simulink model "PassCarModel_RL_config"  (R2024b)
settings: Solver=FixedStepAuto  StartTime=0.0  StopTime=Tf  FixedStep=.001  RelTol=1e-2
StartFcn:
  | %tic
StopFcn:
  | %toc
model workspace (MAT data in the model file):
  AverageTimeInterval = 0.5
  Downshift_Speeds = [9.5625 12.9375 16.3125 19.6875 23.0625 26.4375 29.8125 33.1875 36.5625 39.9375 43.3125 46.6875 ... (28 elements, 4x7)]
  EEC_Counter : Simulink.Parameter (value not decoded)
  EngRevLim = 7000
  FuzzOffset : Simulink.Parameter (value not decoded)
  FuzzRange : Simulink.Parameter (value not decoded)
  Fuzzing : Simulink.Parameter (value not decoded)
  Pedal_Positions = [0.1 0.4 0.5 0.9]
  TrackPoints = [0 36.336 72.672 109.008 145.344 181.68 218.016 254.352 290.688 327.024 363.36 403.196036522 ... (360 elements, 120x3)]
  Upshift_Speeds = [12.9375 16.3125 19.6875 33 26.4375 29.8125 33.1875 52.5 39.9375 43.3125 46.6875 77.25 ... (28 elements, 4x7)]
  VEH : object (value not decoded)
  gradbp : Simulink.Parameter (value not decoded)
  origin : Simulink.Parameter (value not decoded)
  rayDirections = [0 0 0 0 0 0 0 0 0 0 0 0 ... (363 elements, 121x3)]
  rayLengths = [20 20 20 20 20 20 20 20 20 20 20 20 ... (121 elements, 121x1)]
  rayOrigins = [0.5 0.4 0.3 0.2 0.1 0 -0.1 -0.2 -0.3 -0.4 -0.5 0.5 ... (363 elements, 121x3)]
  theta : Simulink.Parameter (value not decoded)
  totalDistance : Simulink.Parameter (value not decoded)
  vel_profile3 : Simulink.Parameter (value not decoded)
  xEast : Simulink.Parameter (value not decoded)
  yNorth : Simulink.Parameter (value not decoded)
symbols that are objects in the model workspace (value not decoded): gradbp, origin, theta, totalDistance, VEH, vel_profile3, xEast, yNorth
undefined symbols (not defined in the file or in its folder): DecelR, DiscIntNeverNeededParam, dspblkCoreblockFVToolHelper, FO_max, FO_min, FR_max, FR_min, gcbh, ODevR, Sim3dSensor, Ts
libraries: simulink x20, dspstat3 x8, autolibutils x6, sim3dgroundtruthsensorlib x2, rllib x1, slpidlib x1, autolibtranscontrolscommon x1, vehdynlibdriver x1, sharedtransform x1, vehdynlibviscommon x1, vehdynlibsens x1
(part 3 of 5)

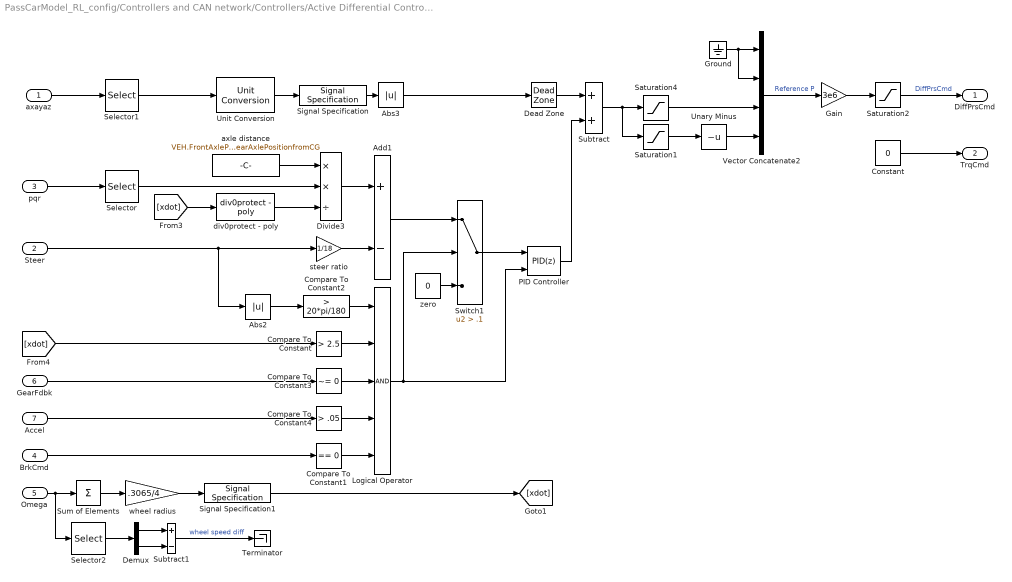
== system PassCarModel_RL_config/Controllers and CAN network/Controllers/Active Differential Control/Rear Diff Controller ==
  axayaz : Inport
  Steer : Inport  Port=2
  pqr : Inport  Port=3
  BrkCmd : Inport  Port=4
  Omega : Inport  Port=5  Unit=rad/s
  GearFdbk : Inport  Port=6
  Accel : Inport  Port=7
  Abs2 : Abs  SaturateOnIntegerOverflow=off
  Abs3 : Abs  ZeroCross=off  SaturateOnIntegerOverflow=off
  Add1 : Sum  Inputs=+-
  Compare To Constant : simulink/Logic and Bit Operations/Compare To Constant  relop=>  const=2.5  OutDataTypeStr=boolean
  Compare To Constant1 : simulink/Logic and Bit Operations/Compare To Constant  relop===  const=0  OutDataTypeStr=boolean
  Compare To Constant2 : simulink/Logic and Bit Operations/Compare To Constant  relop=>  const=20*pi/180  OutDataTypeStr=boolean
  Compare To Constant3 : simulink/Logic and Bit Operations/Compare To Constant  relop=~=  const=0  OutDataTypeStr=boolean
  Compare To Constant4 : simulink/Logic and Bit Operations/Compare To Constant  relop=>  const=.05  OutDataTypeStr=boolean
  Constant : Constant  Value=0
  Dead Zone : DeadZone  ZeroCross=off
  Demux : Demux  Outputs=2
  Divide3 : Product  Inputs=**/
  Gain : Gain  Gain=3e6
  Ground : Ground
  Logical Operator : Logic  Inputs=5  AllPortsSameDT=off  OutDataTypeStr=boolean
  PID Controller : slpidlib/PID Controller  Controller=PID  Form=Parallel  TimeDomain=Discrete-time  UseExternalTs=off  SampleTime=-1  IntegratorMethod=Forward Euler  FilterMethod=Forward Euler  ControllerParametersSource=internal  P=1  I=.05  UseKiTs=off  D=0  UseExternalDerivativeSource=off  N=1  UseFilter=on  TunerSelectOption=Transfer Function Based (PID Tuner App)  ZeroCross=off  InitialConditionSource=internal  InitialConditionForIntegrator=0  InitialConditionForFilter=0  DifferentiatorICPrevScaledInput=0  ExternalReset=either  TrackingMode=off  Kt=1  LimitOutput=on  SatLimitsSource=internal  UpperSaturationLimit=1  LowerSaturationLimit=-1  LinearizeAsGain=on  AntiWindupMode=clamping  Kb=1  LimitIntegrator=off  UpperIntegratorSaturationLimit=inf  LowerIntegratorSaturationLimit=-inf  POutMin=[]  POutMax=[]  IOutMin=[]  IOutMax=[]  DOutMin=[]  DOutMax=[]  NOutMin=[]  NOutMax=[]  SumOutMin=[]  SumOutMax=[]  SaturationOutMin=[]  SaturationOutMax=[]  PParamMin=[]  PParamMax=[]  IParamMin=[]  IParamMax=[]  DParamMin=[]  DParamMax=[]  NParamMin=[]  NParamMax=[]  KbParamMin=[]  KbParamMax=[]  KtParamMin=[]  KtParamMax=[]  KbOutMin=[]  KbOutMax=[]  KtOutMin=[]  KtOutMax=[]  IntegratorOutMin=[]  IntegratorOutMax=[]  FilterOutMin=[]  FilterOutMax=[]  SumI1OutMin=[]  SumI1OutMax=[]  SumI2OutMin=[]  SumI2OutMax=[]  SumI3OutMin=[]  SumI3OutMax=[]  SumI4OutMin=[]  SumI4OutMax=[]  SumDOutMin=[]  SumDOutMax=[]  DifferentiatorOutMin=[]  DifferentiatorOutMax=[]  FilterDiffOutCoefMin=[]  FilterDiffOutCoefMax=[]  ReciprocalOutMin=[]  ReciprocalOutMax=[]  SumDenOutMin=[]  SumDenOutMax=[]  SumNumOutMin=[]  SumNumOutMax=[]  DivideOutMin=[]  DivideOutMax=[]  UdiffTsProdOutMin=[]  UdiffTsProdOutMax=[]  NTsProdOutMin=[]  NTsProdOutMax=[]  UintegralTsProdOutMin=[]  UintegralTsProdOutMax=[]  UngainTsProdOutMin=[]  UngainTsProdOutMax=[]  ClampingZeroOutDataTypeStr=Inherit: Inherit via back propagation  ClampingZeroOutMin=[]  ClampingZeroOutMax=[]  FilterDenConstantOutDataTypeStr=Inherit: Inherit via back propagation  FilterDenConstantOutMin=[]  FilterDenConstantOutMax=[]  PCopyOutDataTypeStr=Inherit: Inherit via back propagation  PCopyOutMin=[]  PCopyOutMax=[]  NCopyOutDataTypeStr=Inherit: Inherit via back propagation  NCopyOutMin=[]  NCopyOutMax=[]  IntegratorContinuousStateAttributes=''  IntegratorStateMustResolveToSignalObject=off  IntegratorRTWStateStorageClass=Auto  FilterContinuousStateAttributes=''  FilterStateMustResolveToSignalObject=off  FilterRTWStateStorageClass=Auto  ParallelPVariant=InternalParameters  IdealPVariant=Disabled  IVariant=InternalParameters  DVariant=InternalParameters  IntegratorVariant=Discrete  SatVariant=Enabled  AWVariant=DiscClampingParallel  PCopyVariant=Disabled  TRVariant=Disabled  FdbkBlocksVariant=Forward  IdealPFdbkVariant=Disabled  SatFdbkVariant=Disabled  DerivativeFilterVariant=ForwardEulerFilter  NVariant=InternalParameters  NCopyVariant=Disabled  FilterICVariant=InternalICsFilter  IntegratorICVariant=InternalICs  ExternalResetVariant=ExternalReset  TRSumVariant=Passthrough  SumFdbkVariant=Disabled  SumVariant=Sum_PID  TsampFilterVariant=InternalTs  TsampNgainVariant=Passthrough  TsampIntegralVariant=Disabled_SignalSpec  ExternalSaturationOutDataTypeStr=Inherit: Same as second input  DerivativeSourceVariant=ErrorSignal  PreIntVariant=InternalPreInt
  Saturation1 : Saturate  UpperLimit=0  LowerLimit=-1  ZeroCross=off
  Saturation2 : Saturate  UpperLimit=5e6  LowerLimit=0  ZeroCross=off
  Saturation4 : Saturate  UpperLimit=1  LowerLimit=0  ZeroCross=off
  Selector : Selector  InputPortWidth=3  IndexOptions=Index vector (dialog)  Indices=[3]  OutputSizes=1
  Selector1 : Selector  InputPortWidth=3  IndexOptions=Index vector (dialog)  Indices=[2]  OutputSizes=1
  Selector2 : Selector  InputPortWidth=4  IndexOptions=Index vector (dialog)  Indices=[3 4]  OutputSizes=1
  Signal Specification : SignalSpecification  Unit=gn
  Signal Specification1 : SignalSpecification  Unit=m/s
  Subtract : Sum
  Subtract1 : Sum  Inputs=+-
  Sum of Elements : Sum  Inputs=+
  Switch1 : Switch  Criteria=u2 > Threshold  Threshold=.1  SaturateOnIntegerOverflow=off  InputSameDT=off
  Terminator : Terminator
  Unary Minus : UnaryMinus
  Unit Conversion : UnitConversion
  Vector Concatenate2 : Concatenate  NumInputs=4
  axle distance : Constant  Value=VEH.FrontAxlePositionfromCG+VEH.RearAxlePositionfromCG
  div0protect - poly : autolibutils/div0protect - poly  thresh=1  ZeroCross1=on  aMode=2
  steer ratio : Gain  Gain=1/18
  wheel radius : Gain  Gain=.3065/4
  zero : Constant  Value=0
  DiffPrsCmd : Outport  VectorParamsAs1DForOutWhenUnconnected=off
  TrqCmd : Outport  Port=2  VectorParamsAs1DForOutWhenUnconnected=off
  wires:
  Vector Concatenate2/1 -> Gain/1  "Reference P"
  Ground/1 -> Vector Concatenate2/2, Vector Concatenate2/1
  Saturation1/1 -> Unary Minus/1
  Gain/1 -> Saturation2/1
  Saturation2/1 -> DiffPrsCmd/1  "DiffPrsCmd"
  Divide3/1 -> Add1/1
  Selector/1 -> Divide3/2
  Logical Operator/1 -> PID Controller/2, Switch1/2
  Switch1/1 -> PID Controller/1
  zero/1 -> Switch1/3
  PID Controller/1 -> Subtract/2
  Add1/1 -> Switch1/1
  axle distance/1 -> Divide3/1
  pqr/1 -> Selector/1
  Compare To Constant2/1 -> Logical Operator/1
  Compare To Constant/1 -> Logical Operator/2
  Abs2/1 -> Compare To Constant2/1
  Steer/1 -> Abs2/1, steer ratio/1
  [xdot] -> Compare To Constant/1
  axayaz/1 -> Selector1/1
  Sum of Elements/1 -> wheel radius/1
  wheel radius/1 -> Signal Specification1/1
  Omega/1 -> Selector2/1, Sum of Elements/1
  Signal Specification1/1 -> [xdot]
  BrkCmd/1 -> Compare To Constant1/1
  GearFdbk/1 -> Compare To Constant3/1
  Compare To Constant3/1 -> Logical Operator/3
  Subtract/1 -> Saturation1/1, Saturation4/1
  Accel/1 -> Compare To Constant4/1
  Compare To Constant4/1 -> Logical Operator/4
  steer ratio/1 -> Add1/2
  Saturation4/1 -> Vector Concatenate2/3
  Selector1/1 -> Unit Conversion/1
  Signal Specification/1 -> Abs3/1
  Abs3/1 -> Dead Zone/1
  Dead Zone/1 -> Subtract/1
  Constant/1 -> TrqCmd/1
  Selector2/1 -> Demux/1
  Demux/1 -> Subtract1/1
  Demux/2 -> Subtract1/2
  Unary Minus/1 -> Vector Concatenate2/4
  Subtract1/1 -> Terminator/1  "wheel speed diff"
  Compare To Constant1/1 -> Logical Operator/5
  Unit Conversion/1 -> Signal Specification/1
  [xdot] -> div0protect - poly/1
  div0protect - poly/1 -> Divide3/3

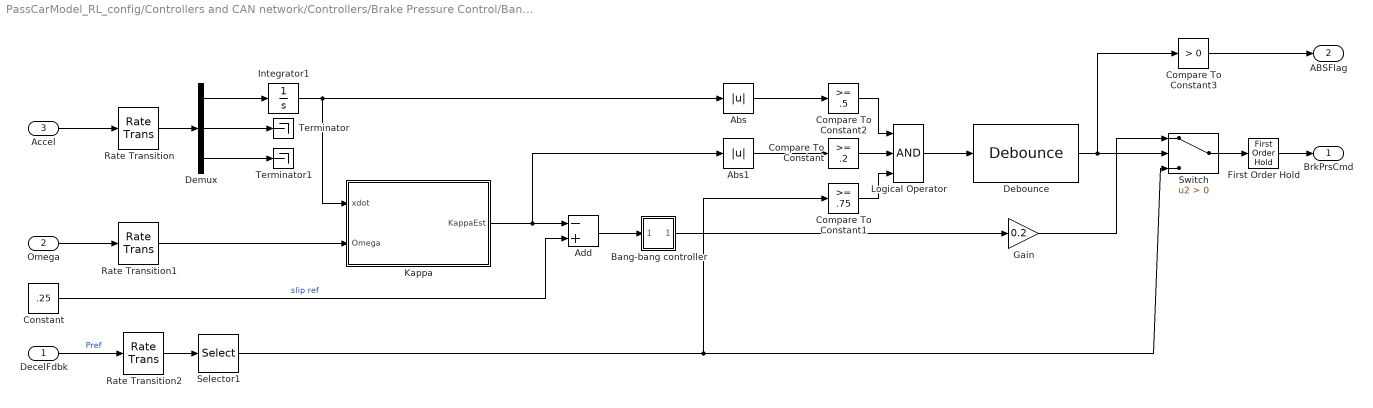
== system PassCarModel_RL_config/Controllers and CAN network/Controllers/Brake Pressure Control/Bang Bang ABS ==
  DecelFdbk : Inport
  Omega : Inport  Port=2
  Accel : Inport  Port=3
  Abs : Abs  SaturateOnIntegerOverflow=off
  Abs1 : Abs  SaturateOnIntegerOverflow=off
  Add : Sum  Inputs=-+
  Bang-bang controller : Subsystem  mask(Sign){}
      mask help: y = sign(x)
      mask Help: Sign Function:\n\t\t\ty = 1 if x > 0\n\t\t\ty = 0 if x = 0\n\t\t\ty = -1 if x < 0
      mask Display: plot(-50,-50,50,50,[-50,50],[0,0],[0,0],[-50,50],[-40,0],[-30,-30],[0,40],[30,30])
  Compare To Constant : simulink/Logic and Bit Operations/Compare To Constant  relop=>=  const=.2  OutDataTypeStr=boolean
  Compare To Constant1 : simulink/Logic and Bit Operations/Compare To Constant  relop=>=  const=.75  OutDataTypeStr=boolean
  Compare To Constant2 : simulink/Logic and Bit Operations/Compare To Constant  relop=>=  const=.5  OutDataTypeStr=boolean
  Compare To Constant3 : simulink/Logic and Bit Operations/Compare To Constant  relop=>  const=0  OutDataTypeStr=boolean  ZeroCross=off
  Constant : Constant  Value=.25
  Debounce : autolibutils/Debounce  DbcOn_Cnts=.1*.001  DbcOff_Cnts=.1*.001  aMode=2
  Demux : Demux  Outputs=3
  First Order Hold : FirstOrderHold  ErrorTolerance=1
  Gain : Gain  Gain=0.2
  Integrator1 : Integrator
  Kappa : Subsystem  TreatAsAtomicUnit=on
  Logical Operator : Logic  Inputs=3  AllPortsSameDT=off  OutDataTypeStr=boolean
  Rate Transition : RateTransition  Deterministic=off  OutPortSampleTime=.001
  Rate Transition1 : RateTransition  Deterministic=off  OutPortSampleTime=.001
  Rate Transition2 : RateTransition  Deterministic=off  OutPortSampleTime=.001
  Selector1 : Selector  InputPortWidth=1  IndexOptions=Index vector (dialog)  Indices=[1 1 1 1]  OutputSizes=1
  Switch : Switch  Criteria=u2 > Threshold  ZeroCross=off  SaturateOnIntegerOverflow=off  InputSameDT=off
  Terminator : Terminator
  Terminator1 : Terminator
  BrkPrsCmd : Outport  VectorParamsAs1DForOutWhenUnconnected=off
  ABSFlag : Outport  Port=2
  wires:
  Bang-bang controller/1(out_1) -> Gain/1
  Add/1 -> Bang-bang controller/1(in_1)
  First Order Hold/1 -> BrkPrsCmd/1
  DecelFdbk/1 -> Rate Transition2/1  "Pref"
  Constant/1 -> Add/2  "slip ref"
  Switch/1 -> First Order Hold/1
  Kappa/1(KappaEst) -> Add/1, Abs1/1
  Logical Operator/1 -> Debounce/1
  Compare To Constant/1 -> Logical Operator/2
  Compare To Constant1/1 -> Logical Operator/3
  Debounce/1 -> Compare To Constant3/1, Switch/2
  Abs/1 -> Compare To Constant2/1
  Compare To Constant2/1 -> Logical Operator/1
  Gain/1 -> Switch/1
  Integrator1/1 -> Kappa/1(xdot), Abs/1
  Demux/2 -> Terminator/1
  Accel/1 -> Rate Transition/1
  Demux/1 -> Integrator1/1
  Rate Transition/1 -> Demux/1
  Demux/3 -> Terminator1/1
  Omega/1 -> Rate Transition1/1
  Rate Transition1/1 -> Kappa/2(Omega)
  Rate Transition2/1 -> Selector1/1
  Compare To Constant3/1 -> ABSFlag/1
  Selector1/1 -> Compare To Constant1/1, Switch/3
  Abs1/1 -> Compare To Constant/1

== system PassCarModel_RL_config/Controllers and CAN network/Controllers/Brake Pressure Control/Five-State ABS and TCS ==
  note: The first order hold block behaves strange: it keeps the ABS flag non-zero after the ABS operation. Its check (if ABS is active) fails elsewhere.
      |
      | The the block is removed
  note: The first order hold block behaves strange: it keeps the ABS flag non-zero after the ABS operation. Its check (if ABS is active) fails elsewhere.
      |
      | The the block is removed
  DecelFdbk : Inport
  Omega : Inport  Port=2
  Accel : Inport  Port=3
  AccelFdbk : Inport  Port=4
  BrkPrs : Inport  Port=5
  ABSCtrlForEach : Subsystem  mask(Five-State ABS Control){Re=0.323, KappaOpt=-0.12, WhlAccelOpt=[-9.8,-9.8,-20,-20], v1=0, v5=0.55, v4=1, a2=-1.5, b=-1.5, A=4.5, a1=3.6, aMode=2}
      mask prompts: Re "Wheel effective radius, Re [m]:"; KappaOpt "Desired wheel slip ratio, KappaOpt [-]:"; WhlAccelOpt "Desired wheel acceleration, WhlAccelOpt [m/s^2]:"; v1 "Braking realease command, v1 [-]:"; v5 "Braking hold command, v5 [-]:"; v4 "Braking add command, v4 [-]:"; a2 "Threshold of State 1, a2 [m/s^2]:"; b "Threshold of State 2, b [m/s^2]:"; A "Threshold of State 3 and 4, A [m/s^2]:"; a1 "Threshold of State 5, a1 [m/s^2]:"
      mask help: This block determines brake pressure varying rate for each wheel once the ABS controller is activated. During ABS control, only wheel speed is directly regulated.
      mask init:
      | [~]=vehdynicon('vehdynblk',gcb);
      mask DialogControl vehParamGroup Prompt: Vehicle Parameter
      mask DialogControl ParameterGroupVar Prompt: Desired Control Parameters
      mask DialogControl Container3 Prompt: Braking Pressure Rates
      mask DialogControl Container4 Prompt: Wheel Acceleration Thresholds
  First Order Hold : FirstOrderHold  ErrorTolerance=.001  AllowContinuousInput=on
  Logical Operator : Logic  Operator=OR  AllPortsSameDT=off  OutDataTypeStr=boolean
  Sum : Sum  Inputs=|++
  Switch : Switch  Criteria=u2 > Threshold  SaturateOnIntegerOverflow=off  InputSameDT=off
  TCSCtrlForEach : Subsystem  mask(Five-State TCS Control){Re=0.323, KappaOpt=0.12, WhlAccelOpt=[11, 11, 11, 11], v1=1.5, v5=-0.5, v4=-1.2, a2=-3, b=-10, A=-11, a1=-9, aMode=2}
      mask prompts: Re "Wheel effective radius, Re [m]:"; KappaOpt "Desired wheel slip ratio, KappaOpt [-]:"; WhlAccelOpt "Desired wheel acceleration, WhlAccelOpt [m/s^2]:"; v1 "Braking pressure rising rate, v1 [-]:"; v5 "Secondary braking pressure declining rate, v5 [-]:"; v4 "Braking pressure declining rate, v4 [-]:"; a2 "Threshold of State 1, a2 [m/s^2]:"; b "Threshold of State 2, b [m/s^2]:"; A "Threshold of State 3 and 4, A [m/s^2]:"; a1 "Threshold of State 5, a1 [m/s^2]:"
      mask help: This block determines brake pressure varying rate for each wheel once the TCS controller is activated. During TCS control, only wheel speed is directly regulated.
      mask init:
      | [~]=vehdynicon('vehdynblk',gcb);
      mask DialogControl vehParamGroup Prompt: Vehicle Parameter
      mask DialogControl ParameterGroupVar Prompt: Desired Control Parameters
      mask DialogControl Container3 Prompt: Braking Pressure Rates
      mask DialogControl Container4 Prompt: Wheel Acceleration Thresholds
  Wheel Accel and Slip Estimator : Subsystem
  BrkPrsCmd : Outport
  ABSFlag : Outport  Port=2  PortDimensions=4
  TCSFlag : Outport  Port=3  PortDimensions=4
  wires:
  Wheel Accel and Slip Estimator/1(<WhlAccel>) -> TCSCtrlForEach/1(WhlAccel), ABSCtrlForEach/2(WhlAccel)
  Wheel Accel and Slip Estimator/2(<Kappa>) -> TCSCtrlForEach/2(WhlSlip), ABSCtrlForEach/3(WhlSlip)
  Wheel Accel and Slip Estimator/3(<xdot>) -> ABSCtrlForEach/4(VehSpd)
  First Order Hold/1 -> BrkPrsCmd/1
  ABSCtrlForEach/2(BrkFlag) -> ABSFlag/1, Logical Operator/1
  Switch/1 -> First Order Hold/1
  TCSCtrlForEach/2(BrkFlag) -> TCSFlag/1, Logical Operator/2
  TCSCtrlForEach/1(BrkCtrl) -> Sum/2
  ABSCtrlForEach/1(BrkCtrl) -> Sum/1
  Sum/1 -> Switch/1
  Logical Operator/1 -> Switch/2
  Accel/1 -> Wheel Accel and Slip Estimator/2(Accel)
  DecelFdbk/1 -> Switch/3, ABSCtrlForEach/1(Pref)
  Omega/1 -> Wheel Accel and Slip Estimator/1(Omega)
  AccelFdbk/1 -> TCSCtrlForEach/3(AccelFdbk)
  BrkPrs/1 -> TCSCtrlForEach/4(PbFdbk)

== system PassCarModel_RL_config/Controllers and CAN network/Controllers/Brake Pressure Control/Open Loop ==
  DecelFdbk : Inport
  Constant : Constant  Value=false
  Constant1 : Constant  Value=false
  Selector : Selector  InputPortWidth=1  IndexOptions=Index vector (dialog)  Indices=[1 1 1 1]  OutputSizes=1
  Selector1 : Selector  InputPortWidth=1  IndexOptions=Index vector (dialog)  Indices=[1 1 1 1]  OutputSizes=1
  Selector2 : Selector  InputPortWidth=1  IndexOptions=Index vector (dialog)  Indices=[1 1 1 1]  OutputSizes=1
  BrkPrsCmd : Outport  VectorParamsAs1DForOutWhenUnconnected=off
  ABSFlag : Outport  Port=2
  TCSFlag : Outport  Port=3
  wires:
  DecelFdbk/1 -> Selector1/1
  Selector1/1 -> BrkPrsCmd/1
  Constant/1 -> Selector/1
  Selector/1 -> ABSFlag/1
  Selector2/1 -> TCSFlag/1
  Constant1/1 -> Selector2/1

== system PassCarModel_RL_config/Controllers and CAN network/Controllers/Brake Pressure Control/Slip control ==
  DecelFdbk : Inport
  Omega : Inport  Port=2
  Accel : Inport  Port=3
  AccelFdbk : Inport  Port=4
  BrkPrs : Inport  Port=5
  ABSCtrlForEach : Subsystem  SystemSampleTime=0.005  mask(Five-State ABS Control){KappaOpt=0, v1=0, v5=0.55, v3=1, a0=-0.5, a1=-0.2, a2=-0.2, a3=-0.05, a4=-0.2, a5=-0.15}
      mask prompts: KappaOpt "Desired wheel slip ratio, KappaOpt [-]:"; v1 "Braking realease command, v1 [-]:"; v5 "Braking hold command, v5 [-]:"; v3 "Braking add command, v3 [-]:"; a0 "Threashold of ABS activation, a0 [-]:"; a1 "Threshold of State 1, a1 [-]:"; a2 "Threshold of State 2, a2 [-]:"; a3 "Threshold of State 3, a3 [-]:"; a4 "Threshold of State 4, a4 [-]:"; a5 "Threshold of State 5, a5 [-]:"
      mask help: This block determines brake pressure varying rate for each wheel once the ABS controller is activated. During ABS control, only wheel speed is directly regulated.
      mask init:
      | [~]=vehdynicon('vehdynblk',gcb);
      mask DialogControl ParameterGroupVar Prompt: Desired Control Parameters
      mask DialogControl Container3 Prompt: Braking Pressure Rates
      mask DialogControl Container4 Prompt: Wheel Slip Thresholds
  First Order Hold : FirstOrderHold  ErrorTolerance=.01  AllowContinuousInput=on
  Logical Operator : Logic  Operator=OR  AllPortsSameDT=off  OutDataTypeStr=boolean
  Sum : Sum  Inputs=|++
  Switch : Switch  Criteria=u2 > Threshold  SaturateOnIntegerOverflow=off  InputSameDT=off
  TCSCtrlForEach : Subsystem  mask(Five-State TCS Control){Re=0.323, KappaOpt=0.12, WhlAccelOpt=[11, 11, 11, 11], v1=1.5, v5=-0.5, v4=-1.2, a2=-6, b=-10, A=-11, a1=-9, aMode=2}
      mask prompts: Re "Wheel effective radius, Re [m]:"; KappaOpt "Desired wheel slip ratio, KappaOpt [-]:"; WhlAccelOpt "Desired wheel acceleration, WhlAccelOpt [m/s^2]:"; v1 "Braking pressure rising rate, v1 [-]:"; v5 "Secondary braking pressure declining rate, v5 [-]:"; v4 "Braking pressure declining rate, v4 [-]:"; a2 "Threshold of State 1, a2 [m/s^2]:"; b "Threshold of State 2, b [m/s^2]:"; A "Threshold of State 3 and 4, A [m/s^2]:"; a1 "Threshold of State 5, a1 [m/s^2]:"
      mask help: This block determines brake pressure varying rate for each wheel once the TCS controller is activated. During TCS control, only wheel speed is directly regulated.
      mask init:
      | [~]=vehdynicon('vehdynblk',gcb);
      mask DialogControl vehParamGroup Prompt: Vehicle Parameter
      mask DialogControl ParameterGroupVar Prompt: Desired Control Parameters
      mask DialogControl Container3 Prompt: Braking Pressure Rates
      mask DialogControl Container4 Prompt: Wheel Acceleration Thresholds
  Wheel Accel and Slip Estimator : Subsystem
  ABSFlag : Outport
  BrkPrsCmd : Outport  Port=2
  TCSFlag : Outport  Port=3
  wires:
  TCSCtrlForEach/2(BrkFlag) -> TCSFlag/1, Logical Operator/2
  Wheel Accel and Slip Estimator/1(<WhlAccel>) -> TCSCtrlForEach/1(WhlAccel)
  ABSCtrlForEach/2(BrkFlag) -> ABSFlag/1, Logical Operator/1
  ABSCtrlForEach/1(BrkCtrl) -> Sum/1
  TCSCtrlForEach/1(BrkCtrl) -> Sum/2
  Switch/1 -> First Order Hold/1
  First Order Hold/1 -> BrkPrsCmd/1
  Wheel Accel and Slip Estimator/2(<Kappa>) -> TCSCtrlForEach/2(WhlSlip), ABSCtrlForEach/2(WhlSlip)
  Omega/1 -> Wheel Accel and Slip Estimator/1(Omega)
  DecelFdbk/1 -> Switch/3, ABSCtrlForEach/1(Pref)
  Sum/1 -> Switch/1
  AccelFdbk/1 -> TCSCtrlForEach/3(AccelFdbk)
  Wheel Accel and Slip Estimator/3(<xdot>) -> ABSCtrlForEach/3(VehSpd)
  BrkPrs/1 -> TCSCtrlForEach/4(PbFdbk)
  Logical Operator/1 -> Switch/2
  Accel/1 -> Wheel Accel and Slip Estimator/2(Accel)

== system PassCarModel_RL_config/Controllers and CAN network/Controllers/ECU/Torque Cmd ==
  note: ABSFlag is a vector of 4 (number of wheels
      | each element should be an integer in [0..5],
      | however it can be a small number instead of zero
  DiffTrqCmd : Inport
  <Accel> : Inport  Port=2
  EngSpd : Inport  Port=3
  ABSFlag : Inport  Port=4
  Acc to Torque Request : Gain  Gain=150
  Constant : Constant  Value=0
  Max : MinMax  Function=max  Inputs=2
  Max of Elements : MinMax  Function=max
  Rev Limiter Control : Subsystem
  Signal Specification : SignalSpecification  Unit=rpm
  Switch : Switch  Criteria=u2 > Threshold  Threshold=0.1  ZeroCross=off  SaturateOnIntegerOverflow=off  InputSameDT=off
  Unit Conversion : UnitConversion
  EngTrqCmd : Outport
  wires:
  Signal Specification/1 -> Rev Limiter Control/2(EngSpd)  "EngSpd"
  Unit Conversion/1 -> Signal Specification/1
  EngSpd/1 -> Unit Conversion/1
  <Accel>/1 -> Acc to Torque Request/1
  Acc to Torque Request/1 -> Rev Limiter Control/1(TrqCmd)
  DiffTrqCmd/1 -> Max/1
  Rev Limiter Control/1(TrqCmdRevLimited) -> Max/2
  Switch/1 -> EngTrqCmd/1
  Max/1 -> Switch/3
  ABSFlag/1 -> Max of Elements/1
  Constant/1 -> Switch/1
  Max of Elements/1 -> Switch/2

== system PassCarModel_RL_config/Controllers and CAN network/Controllers/Transmission Controller/Driver - No Clutch ==
  GearReq : Inport
  Gear : Outport  VectorParamsAs1DForOutWhenUnconnected=off
  wires:
  GearReq/1 -> Gear/1

== system PassCarModel_RL_config/Controllers and CAN network/Controllers/Transmission Controller/PRNDL Controller ==
  Accel : Inport
  BrkCmd : Inport  Port=2
  Omega : Inport  Port=3  Unit=rad/s
  EngSpd : Inport  Port=4  Unit=rad/s
  GearReq : Inport  Port=5
  ABSFlag : Inport  Port=6
  Gain : Gain  Gain=.3065/4
  Logical Operator : Logic  Operator=OR  Inputs=1  AllPortsSameDT=off  OutDataTypeStr=boolean
  Signal Specification1 : SignalSpecification  Unit=m/s
  Sum of Elements : Sum  Inputs=+
  Transmission Controller PRNDL : autolibtranscontrolscommon/Transmission Controller PRNDL  DriveMode=off  GearInit=1  LugSpd=1200  MinUpSpd=2000  tClutchUp=0.5  tClutchDn=0.5  tPark=120  VelUnit=km/hr  UpShSpd="reshape([20    25    30    45    35    45    40    55    40    55    55    65    50    60    65    75    60    65    80    90    70    75   120   150    85    85   150   185  20    25    30    45    35    45    40    55    40    55    55    65    50    60    65    75    60    65    80    90    70    75   120   150    85    85   150   185],4,7,2)"  UpLdBpt=[.1 .4 .75 1]  UpShBpt=1:7  UpPtBpt=[1 2]  DnShfSpd="reshape([10    10    12    15    15    18    18    20    25    25    21    25    30    35    55    55    40    50    65    70    55    65    75    80    75    80    85    95   10    10    12    15    15    18    18    20    25    25    21    25    30    35    55    55    40    50    65    70    55    65    75    80    75    80    85    95],4,7,2)"  DnShSpd=[10 15 25 30 40 55 75; 10 18 25 35 50 65 80; 12 18 21 55 65 75 85; 15 20 25 55 70 80 95]  DnLdBpt=[.1 .4 .75 1]  DnShBpt=2:8  DnPtBpt=[1 2]  POFS=zeros(4,1)  GOFS=zeros(1,7)  Ngears=8  aMode=2
  Gear : Outport  VectorParamsAs1DForOutWhenUnconnected=off
  wires:
  Gain/1 -> Signal Specification1/1
  Omega/1 -> Sum of Elements/1
  Sum of Elements/1 -> Gain/1
  ABSFlag/1 -> Logical Operator/1
  Transmission Controller PRNDL/1 -> Gear/1
  GearReq/1 -> Transmission Controller PRNDL/1  "PRNDL"
  Accel/1 -> Transmission Controller PRNDL/2
  BrkCmd/1 -> Transmission Controller PRNDL/3
  Signal Specification1/1 -> Transmission Controller PRNDL/4
  EngSpd/1 -> Transmission Controller PRNDL/5
  Logical Operator/1 -> Transmission Controller PRNDL/6

== system PassCarModel_RL_config/Controllers and CAN network/Controllers/Transmission Controller/Paddles ==
  Accel : Inport
  EngSpd : Inport  Port=2  Unit=rad/s
  Add1 : Sum  Inputs=+-+
  Current Gear : UnitDelay  SampleTime=-1  HasFrameUpgradeWarning=on
  Data Type Conversion2 : DataTypeConversion  OutDataTypeStr=double  SaturateOnIntegerOverflow=off  RndMeth=Floor
  Debounce : autolibutils/Debounce  DbcOn_Cnts=10  DbcOff_Cnts=10  aMode=aMode
  Debounce1 : autolibutils/Debounce  DbcOn_Cnts=10  DbcOff_Cnts=10  aMode=aMode
  Demux : Demux  Outputs=2
  Detect Increase2 : simulink/Logic and Bit Operations/Detect Increase  vinit=0.0  OutDataTypeStr=boolean
  Logical Operator1 : Logic  Operator=XOR  Inputs=1  AllPortsSameDT=off  OutDataTypeStr=boolean
  Mux : Mux  Inputs=2
  Switch2 : Switch  Criteria=u2 > Threshold  SaturateOnIntegerOverflow=off  InputSameDT=off
  Gear : Outport  VectorParamsAs1DForOutWhenUnconnected=off
  wires:
  Debounce/1 -> Mux/1
  Mux/1 -> Detect Increase2/1
  Logical Operator1/1 -> Switch2/2
  Data Type Conversion2/1 -> Demux/1
  Demux/1 -> Add1/1
  Demux/2 -> Add1/2
  Current Gear/1 -> Add1/3, Switch2/3
  Switch2/1 -> Gear/1, Current Gear/1
  Debounce1/1 -> Mux/2
  Add1/1 -> Switch2/1
  Detect Increase2/1 -> Data Type Conversion2/1, Logical Operator1/1
  EngSpd/1 -> Debounce1/1
  Accel/1 -> Debounce/1

== system PassCarModel_RL_config/Controllers and CAN network/Controllers/Transmission Controller/Transmission Controller ==
  Accel : Inport
  EngSpd : Inport  Port=2  Unit=rad/s
  Omega : Inport  Port=3  Unit=rad/s
  10ms Function-Call Generator : simulink/Ports & Subsystems/Function-Call Generator  sample_time=0.01  numberOfIterations=1  DisallowWideOutput=off
  Data Type Conversion : DataTypeConversion  SaturateOnIntegerOverflow=off  RndMeth=Floor
  First Order Hold : FirstOrderHold  ErrorTolerance=.1
  Rate Transition : RateTransition  Deterministic=off
  Rate Transition1 : RateTransition  Deterministic=off
  Rate Transition2 : RateTransition  Deterministic=off
  Signal Specification : SignalSpecification  Unit=rpm
  TCM : Subsystem
  Unit Conversion : UnitConversion
  Gear : Outport  VectorParamsAs1DForOutWhenUnconnected=off
  wires:
  TCM/1(GearCmd) -> Data Type Conversion/1
  Rate Transition/1 -> TCM/1(AccCmd)
  10ms Function-Call Generator/1 -> TCM/Trigger
  Accel/1 -> Rate Transition/1
  Omega/1 -> Rate Transition2/1
  Rate Transition1/1 -> TCM/2(EngSpd)
  First Order Hold/1 -> Gear/1
  Unit Conversion/1 -> Signal Specification/1
  Signal Specification/1 -> Rate Transition1/1  "EngSpd"
  EngSpd/1 -> Unit Conversion/1
  Data Type Conversion/1 -> First Order Hold/1
  Rate Transition2/1 -> TCM/3(Omega)

== system PassCarModel_RL_config/Controllers and CAN network/Gateway/BC-Filter/FilterABSTCSFlags ==
  In1 : Inport
  In2 : Inport  Port=2
  Out1 : Outport
  Out2 : Outport  Port=2
  wires:
  In1/1 -> Out1/1
  In2/1 -> Out2/1

== system PassCarModel_RL_config/Controllers and CAN network/Gateway/BC-Filter/FilterBrkPrs ==
  In1 : Inport
  Out1 : Outport
  wires:
  In1/1 -> Out1/1

== system PassCarModel_RL_config/Controllers and CAN network/Gateway/BC-Filter/FilterBrkPrsCmd ==
  In1 : Inport
  Out1 : Outport
  wires:
  In1/1 -> Out1/1

== system PassCarModel_RL_config/Controllers and CAN network/Gateway/BC-Filter/FilterWheelSpeed ==
  VehicleSpeed : Inport
  Omega : Inport  Port=2
  PrpShftSpd : Inport  Port=3
  OmegaFuzz : Inport  Port=4
  AllCombinationCounted : Subsystem
  Bus Creator : BusCreator  Inputs=4
  Data Type Conversion : DataTypeConversion  SaturateOnIntegerOverflow=off  RndMeth=Floor
  Data Type Conversion{1..7} (7 alike) : DataTypeConversion  OutDataTypeStr=double  SaturateOnIntegerOverflow=off  RndMeth=Floor
  MATLAB Function : MATLAB Function  TreatAsAtomicUnit=on
  Signal holder : Subsystem
  Terminator{,2..5} (5 alike) : Terminator
  OmegaFiltered : Outport
  wires:
  MATLAB Function/2(diff_ratio) -> Data Type Conversion3/1  "diff_ratio"
  MATLAB Function/4(y1) -> Data Type Conversion5/1  "RearAxle_WS_check"
  MATLAB Function/1(y) -> Data Type Conversion7/1  "Decision"
  MATLAB Function/3(wheel_speed_max) -> Data Type Conversion4/1  "wheel_speed_max"
  MATLAB Function/5(y2) -> Data Type Conversion6/1  "VehSpeed_WS_Check"
  VehicleSpeed/1 -> Data Type Conversion/1
  PrpShftSpd/1 -> Data Type Conversion1/1
  OmegaFuzz/1 -> AllCombinationCounted/2(Input2)
  AllCombinationCounted/2(Input1 && ~Input2) -> Bus Creator/2  "RealAccept"
  AllCombinationCounted/1(Input1 && Input2) -> Bus Creator/1  "FuzzAccept"
  AllCombinationCounted/3(~Input1 && Input2) -> Bus Creator/3  "FuzzReject"
  AllCombinationCounted/4(~Input1 && ~Input2) -> Bus Creator/4  "RealReject"
  Bus Creator/1 -> Terminator/1  "FilterEfficiency"
  Omega/1 -> Data Type Conversion2/1, Signal holder/1(SignalIn)  "OmegaRaw"
  Signal holder/1(SignalOut) -> OmegaFiltered/1  "OmegaFiltered"
  Data Type Conversion/1 -> MATLAB Function/3(VehSpeed)
  Data Type Conversion1/1 -> MATLAB Function/2(OutputShaftSpeed)
  Data Type Conversion2/1 -> MATLAB Function/1(WheelSpeeds)
  Data Type Conversion3/1 -> Terminator2/1
  Data Type Conversion4/1 -> Terminator3/1
  Data Type Conversion5/1 -> Terminator4/1
  Data Type Conversion6/1 -> Terminator5/1
  Data Type Conversion7/1 -> AllCombinationCounted/1(Input1), Signal holder/2(Condition)

== system PassCarModel_RL_config/Vehicle with driver and environment/Environment/Ground Feedback/3D Engine ==
  Friction : Inport
  VehFdbk : Inport  Port=2
  3D Engine Source : Subsystem  Variant=on  VariantControl=Choice  mask(Terrain Source){terrType=Single point}
      mask prompts: terrType "Terrain feedback type:"
      mask help:
      | This variant subsystem provides the option for:
      | - a single point of contact for each wheel with minimal post-processing ideal for smooth surfaces and maximum run-time performance.
      | - multiple points of contact per wheel which may be used when interested in non-smooth terrain at a higher computational cost.
      mask TypeOptions terrType: Single point | Multiple points
  Bus Creator2 : BusCreator  Inputs=4
  Bus Creator3 : BusCreator  Inputs=3
  Demux1 : Demux
  Signal Specification1 : SignalSpecification  Unit=1
  Ground : Outport  VectorParamsAs1DForOutWhenUnconnected=off
  wires:
  Signal Specification1/1 -> Demux1/1
  Demux1/1 -> Bus Creator2/1  "mu_FL"
  Demux1/3 -> Bus Creator2/3  "mu_RL"
  Demux1/4 -> Bus Creator2/4  "mu_RR"
  Demux1/2 -> Bus Creator2/2  "mu_FR"
  Bus Creator2/1 -> Bus Creator3/3  "mu"
  Bus Creator3/1 -> Ground/1
  Friction/1 -> Signal Specification1/1
  VehFdbk/1 -> 3D Engine Source/1(VehFdbk)
  3D Engine Source/1(z) -> Bus Creator3/1  "z"
  3D Engine Source/2(DCM) -> Bus Creator3/2  "DCM"

== system PassCarModel_RL_config/Vehicle with driver and environment/Environment/Ground Feedback/Constant ==
  Friction : Inport
  Bus Creator : BusCreator  Inputs=4
  Bus Creator2 : BusCreator  Inputs=4
  Bus Creator3 : BusCreator  Inputs=3
  Constant1 : Constant  Value=zeros(4,1)
  Constant4 : Constant  Value=repmat(eye(3),1,1,4)
  Demux : Demux
  Demux1 : Demux
  Signal Specification : SignalSpecification  Unit=m
  Signal Specification1 : SignalSpecification  Unit=1
  Ground : Outport  VectorParamsAs1DForOutWhenUnconnected=off
  wires:
  Constant1/1 -> Signal Specification/1
  Signal Specification/1 -> Demux/1
  Demux/4 -> Bus Creator/4  "G_RR_z"
  Demux/1 -> Bus Creator/1  "G_FL_z"
  Demux/3 -> Bus Creator/3  "G_RL_z"
  Demux/2 -> Bus Creator/2  "G_FR_z"
  Bus Creator/1 -> Bus Creator3/1  "z"
  Demux1/3 -> Bus Creator2/3  "mu_RL"
  Demux1/4 -> Bus Creator2/4  "mu_RR"
  Demux1/1 -> Bus Creator2/1  "mu_FL"
  Demux1/2 -> Bus Creator2/2  "mu_FR"
  Bus Creator2/1 -> Bus Creator3/3  "mu"
  Friction/1 -> Signal Specification1/1
  Signal Specification1/1 -> Demux1/1
  Bus Creator3/1 -> Ground/1
  Constant4/1 -> Bus Creator3/2  "DCM"

== system PassCarModel_RL_config/Vehicle with driver and environment/Environment/Road Track Friction/2D Lookup Tbl for Scaling Fctr (Lambda) ==
  XWhl : Inport  Partition=on  PartitionDimension=1  PartitionWidth=1  PartitionOffset=0
  YWhl : Inport  Port=2  Partition=on  PartitionDimension=1  PartitionWidth=1  PartitionOffset=0
  XBpt : Inport  Port=3
  YBpt : Inport  Port=4
  2-D Lookup Table : Lookup_n-D  BreakpointsForDimension1Source=Input port  BreakpointsForDimension1=xbr  BreakpointsForDimension2Source=Input port  BreakpointsForDimension2=ybr  BeginIndexSearchUsingPreviousIndexResult=on  Table=mutable  ExtrapMethod=Clip  InternalRulePriority=Speed  RndMeth=Simplest
      settings: InputPortMap=u0,u1,p5,p7
  For Each : ForEach  DisableCoverage=on
  Lambda for each whl : Outport  ConcatenationDimension=1
  wires:
  XWhl/1 -> 2-D Lookup Table/1
  YWhl/1 -> 2-D Lookup Table/2
  2-D Lookup Table/1 -> Lambda for each whl/1
  XBpt/1 -> 2-D Lookup Table/3
  YBpt/1 -> 2-D Lookup Table/4

== system PassCarModel_RL_config/Vehicle with driver and environment/Environment/Road Track Friction/Creating Inertial Frm Bpt ==
  XCg : Inport
  YCg : Inport  Port=2
  Enable : EnablePort
  Add : Sum
  Add1 : Sum
  Constant1 : Constant  Value=ybr
  Constant3 : Constant  Value=xbr
  XBpt : Outport
  YBpt : Outport  Port=2
  wires:
  Add/1 -> XBpt/1
  Constant1/1 -> Add1/1
  Add1/1 -> YBpt/1
  Constant3/1 -> Add/2
  YCg/1 -> Add1/2
  XCg/1 -> Add/1

== system PassCarModel_RL_config/Vehicle with driver and environment/Environment/Road Track Friction/En at t = 0 ==
  Clock1 : Clock
  Compare To Zero : simulink/Logic and Bit Operations/Compare To Zero  relop===  OutDataTypeStr=boolean
  Constant : Constant
  Constant2 : Constant  Value=0
  Switch1 : Switch  Criteria=u2 > Threshold  SaturateOnIntegerOverflow=off  InputSameDT=off
  Out1 : Outport
  wires:
  Clock1/1 -> Compare To Zero/1
  Constant2/1 -> Switch1/3
  Constant/1 -> Switch1/1
  Switch1/1 -> Out1/1
  Compare To Zero/1 -> Switch1/2

== system PassCarModel_RL_config/Vehicle with driver and environment/Passenger Vehicle/Pedal Cluster and Cabin/Brake Pedal ==
  DecelCmd : Inport
  Constant1 : Constant  Value=-20
  Dead Zone1 : DeadZone  LowerValue=0  UpperValue=.01  ZeroCross=off
  Gain3 : Gain  Gain=40
  Integrator2 : Integrator  LimitOutput=on  UpperSaturationLimit=1  LowerSaturationLimit=0
  Switch1 : Switch  Criteria=u2 > Threshold  Threshold=.1  SaturateOnIntegerOverflow=off  InputSameDT=off
  DecelFdbk : Outport
  wires:
  Dead Zone1/1 -> Switch1/2, Gain3/1
  Constant1/1 -> Switch1/3
  Integrator2/1 -> DecelFdbk/1
  Gain3/1 -> Switch1/1
  Switch1/1 -> Integrator2/1
  DecelCmd/1 -> Dead Zone1/1

== system PassCarModel_RL_config/Controllers and CAN network/CAN/BrakeController/EBC1/ControlFlag ==
  note: 4 bit unsigned
      | factor - 1
      | offset - 0
      | min - 0
      | max - 15
      | unit - N/A
  In1 : Inport
  Memory : Memory
  Zero-Order Hold : ZeroOrderHold  SampleTime=0.005
  fix point : DataTypeConversion  OutMin=0  OutMax=15  OutDataTypeStr=fixdt(0,4,1,0)  SaturateOnIntegerOverflow=off  RndMeth=Floor
  Out2 : Outport
  wires:
  In1/1 -> Zero-Order Hold/1
  Memory/1 -> Out2/1
  fix point/1 -> Memory/1
  Zero-Order Hold/1 -> fix point/1

== system PassCarModel_RL_config/Controllers and CAN network/CAN/BrakeController/EBC1/ControlFlag1 ==
  note: 4 bit unsigned
      | factor - 1
      | offset - 0
      | min - 0
      | max - 15
      | unit - N/A
  In1 : Inport
  Memory : Memory
  Zero-Order Hold : ZeroOrderHold  SampleTime=0.005
  fix point : DataTypeConversion  OutMin=0  OutMax=15  OutDataTypeStr=fixdt(0,4,1,0)  SaturateOnIntegerOverflow=off  RndMeth=Floor
  Out2 : Outport
  wires:
  In1/1 -> Zero-Order Hold/1
  Memory/1 -> Out2/1
  fix point/1 -> Memory/1
  Zero-Order Hold/1 -> fix point/1

== system PassCarModel_RL_config/Controllers and CAN network/CAN/BrakeController/EBC1/ControlFlag2 ==
  note: 4 bit unsigned
      | factor - 1
      | offset - 0
      | min - 0
      | max - 15
      | unit - N/A
  In1 : Inport
  Memory : Memory
  Zero-Order Hold : ZeroOrderHold  SampleTime=0.005
  fix point : DataTypeConversion  OutMin=0  OutMax=15  OutDataTypeStr=fixdt(0,4,1,0)  SaturateOnIntegerOverflow=off  RndMeth=Floor
  Out2 : Outport
  wires:
  In1/1 -> Zero-Order Hold/1
  Memory/1 -> Out2/1
  fix point/1 -> Memory/1
  Zero-Order Hold/1 -> fix point/1

== system PassCarModel_RL_config/Controllers and CAN network/CAN/BrakeController/EBC1/ControlFlag3 ==
  note: 4 bit unsigned
      | factor - 1
      | offset - 0
      | min - 0
      | max - 15
      | unit - N/A
  In1 : Inport
  Memory : Memory
  Zero-Order Hold : ZeroOrderHold  SampleTime=0.005
  fix point : DataTypeConversion  OutMin=0  OutMax=15  OutDataTypeStr=fixdt(0,4,1,0)  SaturateOnIntegerOverflow=off  RndMeth=Floor
  Out2 : Outport
  wires:
  In1/1 -> Zero-Order Hold/1
  Memory/1 -> Out2/1
  fix point/1 -> Memory/1
  Zero-Order Hold/1 -> fix point/1

== system PassCarModel_RL_config/Controllers and CAN network/CAN/BrakeController/EBC1/ControlFlag4 ==
  note: 4 bit unsigned
      | factor - 1
      | offset - 0
      | min - 0
      | max - 15
      | unit - N/A
  In1 : Inport
  Memory : Memory
  Zero-Order Hold : ZeroOrderHold  SampleTime=0.005
  fix point : DataTypeConversion  OutMin=0  OutMax=15  OutDataTypeStr=fixdt(0,4,1,0)  SaturateOnIntegerOverflow=off  RndMeth=Floor
  Out2 : Outport
  wires:
  In1/1 -> Zero-Order Hold/1
  Memory/1 -> Out2/1
  fix point/1 -> Memory/1
  Zero-Order Hold/1 -> fix point/1

== system PassCarModel_RL_config/Controllers and CAN network/CAN/BrakeController/EBC1/ControlFlag5 ==
  note: 4 bit unsigned
      | factor - 1
      | offset - 0
      | min - 0
      | max - 15
      | unit - N/A
  In1 : Inport
  Memory : Memory
  Zero-Order Hold : ZeroOrderHold  SampleTime=0.005
  fix point : DataTypeConversion  OutMin=0  OutMax=15  OutDataTypeStr=fixdt(0,4,1,0)  SaturateOnIntegerOverflow=off  RndMeth=Floor
  Out2 : Outport
  wires:
  In1/1 -> Zero-Order Hold/1
  Memory/1 -> Out2/1
  fix point/1 -> Memory/1
  Zero-Order Hold/1 -> fix point/1

== system PassCarModel_RL_config/Controllers and CAN network/CAN/BrakeController/EBC1/ControlFlag6 ==
  note: 4 bit unsigned
      | factor - 1
      | offset - 0
      | min - 0
      | max - 15
      | unit - N/A
  In1 : Inport
  Memory : Memory
  Zero-Order Hold : ZeroOrderHold  SampleTime=0.005
  fix point : DataTypeConversion  OutMin=0  OutMax=15  OutDataTypeStr=fixdt(0,4,1,0)  SaturateOnIntegerOverflow=off  RndMeth=Floor
  Out2 : Outport
  wires:
  In1/1 -> Zero-Order Hold/1
  Memory/1 -> Out2/1
  fix point/1 -> Memory/1
  Zero-Order Hold/1 -> fix point/1

== system PassCarModel_RL_config/Controllers and CAN network/CAN/BrakeController/EBC1/ControlFlag7 ==
  note: 4 bit unsigned
      | factor - 1
      | offset - 0
      | min - 0
      | max - 15
      | unit - N/A
  In1 : Inport
  Memory : Memory
  Zero-Order Hold : ZeroOrderHold  SampleTime=0.005
  fix point : DataTypeConversion  OutMin=0  OutMax=15  OutDataTypeStr=fixdt(0,4,1,0)  SaturateOnIntegerOverflow=off  RndMeth=Floor
  Out2 : Outport
  wires:
  In1/1 -> Zero-Order Hold/1
  Memory/1 -> Out2/1
  fix point/1 -> Memory/1
  Zero-Order Hold/1 -> fix point/1

== system PassCarModel_RL_config/Controllers and CAN network/CAN/BrakeController/EBC2/BrakePressure ==
  note: 16 bit unsigned
      | factor - 1
      | offset - 0
      | min - 0
      | max - 65535
      | unit - kPa
  In1 : Inport
  Memory : Memory
  Zero-Order Hold : ZeroOrderHold  SampleTime=0.005
  fix point : DataTypeConversion  OutMin=0  OutMax=65535  OutDataTypeStr=fixdt(0,16,1,0)  SaturateOnIntegerOverflow=off  RndMeth=Floor
  Out2 : Outport
  wires:
  Zero-Order Hold/1 -> fix point/1
  fix point/1 -> Memory/1
  Memory/1 -> Out2/1
  In1/1 -> Zero-Order Hold/1

== system PassCarModel_RL_config/Controllers and CAN network/CAN/BrakeController/EBC2/BrakePressure1 ==
  note: 16 bit unsigned
      | factor - 1
      | offset - 0
      | min - 0
      | max - 65535
      | unit - kPa
  In1 : Inport
  Memory : Memory
  Zero-Order Hold : ZeroOrderHold  SampleTime=0.005
  fix point : DataTypeConversion  OutMin=0  OutMax=65535  OutDataTypeStr=fixdt(0,16,1,0)  SaturateOnIntegerOverflow=off  RndMeth=Floor
  Out2 : Outport
  wires:
  Zero-Order Hold/1 -> fix point/1
  fix point/1 -> Memory/1
  Memory/1 -> Out2/1
  In1/1 -> Zero-Order Hold/1

== system PassCarModel_RL_config/Controllers and CAN network/CAN/BrakeController/EBC2/BrakePressure2 ==
  note: 16 bit unsigned
      | factor - 1
      | offset - 0
      | min - 0
      | max - 65535
      | unit - kPa
  In1 : Inport
  Memory : Memory
  Zero-Order Hold : ZeroOrderHold  SampleTime=0.005
  fix point : DataTypeConversion  OutMin=0  OutMax=65535  OutDataTypeStr=fixdt(0,16,1,0)  SaturateOnIntegerOverflow=off  RndMeth=Floor
  Out2 : Outport
  wires:
  Zero-Order Hold/1 -> fix point/1
  fix point/1 -> Memory/1
  Memory/1 -> Out2/1
  In1/1 -> Zero-Order Hold/1

== system PassCarModel_RL_config/Controllers and CAN network/CAN/BrakeController/EBC2/BrakePressure3 ==
  note: 16 bit unsigned
      | factor - 1
      | offset - 0
      | min - 0
      | max - 65535
      | unit - kPa
  In1 : Inport
  Memory : Memory
  Zero-Order Hold : ZeroOrderHold  SampleTime=0.005
  fix point : DataTypeConversion  OutMin=0  OutMax=65535  OutDataTypeStr=fixdt(0,16,1,0)  SaturateOnIntegerOverflow=off  RndMeth=Floor
  Out2 : Outport
  wires:
  Zero-Order Hold/1 -> fix point/1
  fix point/1 -> Memory/1
  Memory/1 -> Out2/1
  In1/1 -> Zero-Order Hold/1

== system PassCarModel_RL_config/Controllers and CAN network/CAN/BrakeController/EBC3/BrakePressureCmd ==
  note: 8 bit unsigned
      | factor - 0.01
      | offset - 0
      | min - 0
      | max - 2.55
      | unit - N/A
  In1 : Inport
  Memory : Memory
  Zero-Order Hold : ZeroOrderHold  SampleTime=0.005
  fix point : DataTypeConversion  OutMin=0  OutMax=2.55  OutDataTypeStr=fixdt(0,8,0.01,0)  SaturateOnIntegerOverflow=off  RndMeth=Floor
  Out2 : Outport
  wires:
  In1/1 -> Zero-Order Hold/1
  Memory/1 -> Out2/1
  fix point/1 -> Memory/1
  Zero-Order Hold/1 -> fix point/1

== system PassCarModel_RL_config/Controllers and CAN network/CAN/BrakeController/EBC3/BrakePressureCmd1 ==
  note: 8 bit unsigned
      | factor - 0.01
      | offset - 0
      | min - 0
      | max - 2.55
      | unit - N/A
  In1 : Inport
  Memory : Memory
  Zero-Order Hold : ZeroOrderHold  SampleTime=0.005
  fix point : DataTypeConversion  OutMin=0  OutMax=2.55  OutDataTypeStr=fixdt(0,8,0.01,0)  SaturateOnIntegerOverflow=off  RndMeth=Floor
  Out2 : Outport
  wires:
  In1/1 -> Zero-Order Hold/1
  Memory/1 -> Out2/1
  fix point/1 -> Memory/1
  Zero-Order Hold/1 -> fix point/1

== system PassCarModel_RL_config/Controllers and CAN network/CAN/BrakeController/EBC3/BrakePressureCmd2 ==
  note: 8 bit unsigned
      | factor - 0.01
      | offset - 0
      | min - 0
      | max - 2.55
      | unit - N/A
  In1 : Inport
  Memory : Memory
  Zero-Order Hold : ZeroOrderHold  SampleTime=0.005
  fix point : DataTypeConversion  OutMin=0  OutMax=2.55  OutDataTypeStr=fixdt(0,8,0.01,0)  SaturateOnIntegerOverflow=off  RndMeth=Floor
  Out2 : Outport
  wires:
  In1/1 -> Zero-Order Hold/1
  Memory/1 -> Out2/1
  fix point/1 -> Memory/1
  Zero-Order Hold/1 -> fix point/1

== system PassCarModel_RL_config/Controllers and CAN network/CAN/BrakeController/EBC3/BrakePressureCmd3 ==
  note: 8 bit unsigned
      | factor - 0.01
      | offset - 0
      | min - 0
      | max - 2.55
      | unit - N/A
  In1 : Inport
  Memory : Memory
  Zero-Order Hold : ZeroOrderHold  SampleTime=0.005
  fix point : DataTypeConversion  OutMin=0  OutMax=2.55  OutDataTypeStr=fixdt(0,8,0.01,0)  SaturateOnIntegerOverflow=off  RndMeth=Floor
  Out2 : Outport
  wires:
  In1/1 -> Zero-Order Hold/1
  Memory/1 -> Out2/1
  fix point/1 -> Memory/1
  Zero-Order Hold/1 -> fix point/1

== system PassCarModel_RL_config/Controllers and CAN network/CAN/BrakeController/EBC4/Noise Mixer ==
  Enabled : Inport
  Noise : Inport  Port=2
  Constant : Constant  Value=3
  Counter Limited : simulink/Sources/Counter Limited  uplimit=4  tsamp=0.001
  Delay : Delay  DelayLength=3  InitialCondition=0
  Logical Operator : Logic  Operator=OR  AllPortsSameDT=off  OutDataTypeStr=boolean
  Logical Operator1 : Logic  Operator=NOT  AllPortsSameDT=off  OutDataTypeStr=boolean
  Relational Operator : RelationalOperator  Operator=<=  OutDataTypeStr=boolean  RndMeth=Simplest  InputSameDT=off
  WheelSpeed2 : Subsystem
  Zero-Order Hold : ZeroOrderHold  SampleTime=0.005
  trigger : Outport
  noise : Outport  Port=2
  wires:
  Relational Operator/1 -> Logical Operator/2, WheelSpeed2/Trigger  "GenerateTrigger"
  Zero-Order Hold/1 -> WheelSpeed2/1(In1)
  Counter Limited/1 -> Delay/1
  Noise/1 -> Zero-Order Hold/1
  WheelSpeed2/1(Out2) -> noise/1  "noise"
  Delay/1 -> Relational Operator/2
  Constant/1 -> Relational Operator/1
  Enabled/1 -> Logical Operator1/1
  Logical Operator/1 -> trigger/1  "trigger"
  Logical Operator1/1 -> Logical Operator/1

== system PassCarModel_RL_config/Controllers and CAN network/CAN/BrakeController/EBC4/WheelSpeed ==
  note: 15 bit unsigned
      | factor - 0.005
      | offset - 0
      | min - 0
      | max - 163.835
      | unit - km/h
  In1 : Inport
  Memory : Memory
  Zero-Order Hold : ZeroOrderHold  SampleTime=0.005
  fix point : DataTypeConversion  OutMin=0  OutMax=163.835  OutDataTypeStr=fixdt(0,15,0.005,0)  SaturateOnIntegerOverflow=off  RndMeth=Floor
  Out2 : Outport
  wires:
  Zero-Order Hold/1 -> fix point/1
  fix point/1 -> Memory/1
  Memory/1 -> Out2/1
  In1/1 -> Zero-Order Hold/1

== system PassCarModel_RL_config/Controllers and CAN network/CAN/BrakeController/EBC4/WheelSpeed1 ==
  note: 15 bit unsigned
      | factor - 0.005
      | offset - 0
      | min - 0
      | max - 163.835
      | unit - km/h
  In1 : Inport
  Memory : Memory
  Zero-Order Hold : ZeroOrderHold  SampleTime=0.005
  fix point : DataTypeConversion  OutMin=0  OutMax=163.835  OutDataTypeStr=fixdt(0,15,0.005,0)  SaturateOnIntegerOverflow=off  RndMeth=Floor
  Out2 : Outport
  wires:
  Zero-Order Hold/1 -> fix point/1
  fix point/1 -> Memory/1
  Memory/1 -> Out2/1
  In1/1 -> Zero-Order Hold/1

== system PassCarModel_RL_config/Controllers and CAN network/CAN/BrakeController/EBC4/WheelSpeed2 ==
  note: 15 bit unsigned
      | factor - 0.005
      | offset - 0
      | min - 0
      | max - 163.835
      | unit - km/h
  In1 : Inport
  Memory : Memory
  Zero-Order Hold : ZeroOrderHold  SampleTime=0.005
  fix point : DataTypeConversion  OutMin=0  OutMax=163.835  OutDataTypeStr=fixdt(0,15,0.005,0)  SaturateOnIntegerOverflow=off  RndMeth=Floor
  Out2 : Outport
  wires:
  Zero-Order Hold/1 -> fix point/1
  fix point/1 -> Memory/1
  Memory/1 -> Out2/1
  In1/1 -> Zero-Order Hold/1

== system PassCarModel_RL_config/Controllers and CAN network/CAN/BrakeController/EBC4/WheelSpeed3 ==
  note: 15 bit unsigned
      | factor - 0.005
      | offset - 0
      | min - 0
      | max - 163.835
      | unit - km/h
  In1 : Inport
  Memory : Memory
  Zero-Order Hold : ZeroOrderHold  SampleTime=0.005
  fix point : DataTypeConversion  OutMin=0  OutMax=163.835  OutDataTypeStr=fixdt(0,15,0.005,0)  SaturateOnIntegerOverflow=off  RndMeth=Floor
  Out2 : Outport
  wires:
  Zero-Order Hold/1 -> fix point/1
  fix point/1 -> Memory/1
  Memory/1 -> Out2/1
  In1/1 -> Zero-Order Hold/1

== system PassCarModel_RL_config/Controllers and CAN network/CAN/CentralController/ECC1/ControlSignal2 ==
  note: 8 bit unsigned
      | factor - 0.005
      | offset - 0
      | min - 0
      | max - 1.275
      | unit - %
  In1 : Inport
  Memory : Memory
  Zero-Order Hold : ZeroOrderHold  SampleTime=0.005
  fix point : DataTypeConversion  OutMin=0  OutMax=1.275  OutDataTypeStr=fixdt(0,8,0.005,0)  SaturateOnIntegerOverflow=off  RndMeth=Floor
  Out2 : Outport
  wires:
  Zero-Order Hold/1 -> fix point/1
  fix point/1 -> Memory/1
  Memory/1 -> Out2/1
  In1/1 -> Zero-Order Hold/1

== system PassCarModel_RL_config/Controllers and CAN network/CAN/CentralController/ECC1/ControlSignal3 ==
  note: 8 bit unsigned
      | factor - 0.005
      | offset - 0
      | min - 0
      | max - 1.275
      | unit - %
  In1 : Inport
  Memory : Memory
  Zero-Order Hold : ZeroOrderHold  SampleTime=0.005
  fix point : DataTypeConversion  OutMin=0  OutMax=1.275  OutDataTypeStr=fixdt(0,8,0.005,0)  SaturateOnIntegerOverflow=off  RndMeth=Floor
  Out2 : Outport
  wires:
  Zero-Order Hold/1 -> fix point/1
  fix point/1 -> Memory/1
  Memory/1 -> Out2/1
  In1/1 -> Zero-Order Hold/1

== system PassCarModel_RL_config/Controllers and CAN network/CAN/CentralController/ECC1/Gear1 ==
  note: 8 bit unsigned
      | factor - 1
      | offset - 0
      | min - -125
      | max - 125
      | unit - deg
  In1 : Inport
  Memory : Memory
  Zero-Order Hold : ZeroOrderHold  SampleTime=0.005
  fix point : DataTypeConversion  OutMin=-125  OutMax=125  OutDataTypeStr=fixdt(0,8,1,-125)  SaturateOnIntegerOverflow=off  RndMeth=Floor
  Out2 : Outport
  wires:
  Zero-Order Hold/1 -> fix point/1
  fix point/1 -> Memory/1
  Memory/1 -> Out2/1
  In1/1 -> Zero-Order Hold/1

== system PassCarModel_RL_config/Controllers and CAN network/CAN/CentralController/ECC1/SteeringWheelPos1 ==
  note: 16 bit unsigned
      | factor - 0.04
      | offset - -1300
      | min - -1300
      | max - 1321.4
      | unit - deg
  In1 : Inport
  Memory : Memory
  Zero-Order Hold : ZeroOrderHold  SampleTime=0.005
  fix point : DataTypeConversion  OutMin=-1300  OutMax=1320.4  OutDataTypeStr=fixdt(0,16,0.04,-1300)  SaturateOnIntegerOverflow=off  RndMeth=Floor
  Out2 : Outport
  wires:
  In1/1 -> Zero-Order Hold/1
  Memory/1 -> Out2/1
  fix point/1 -> Memory/1
  Zero-Order Hold/1 -> fix point/1
